simulink model "DiscreteSF_obs"  (R2019b)
settings: Solver=VariableStepAuto  StartTime=0.0  StopTime=10.0  RelTol=1e-3
values from neighbouring files (symbols this model uses):
  th1 = 0.85    [AP_TimeDelay.m]    (also in SmithControl.m; TimeDelayParameters.m = 0.32; positivity_matrix.m; rscale.m)
  th2 = 50    [AP_TimeDelay.m]    (also in SmithControl.m; TimeDelayParameters.m; positivity_matrix.m; rscale.m)
  th3 = 60    [AP_TimeDelay.m]    (also in SmithControl.m; TimeDelayParameters.m = 70; positivity_matrix.m; rscale.m)
undefined symbols (not defined in the file or in its folder): A3, B3, C_obs, D_obs, F3, L_obs
libraries: dspsrcs4 x1
settings Model: Creator=akshita_jain  LastModifiedBy=akshita_jain

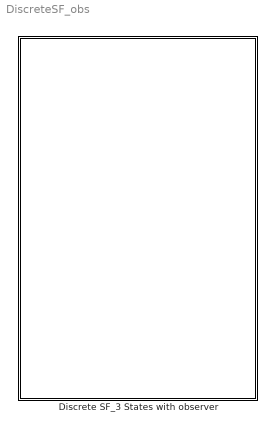
== system DiscreteSF_obs ==
  Discrete SF_3 States with observer : Subsystem

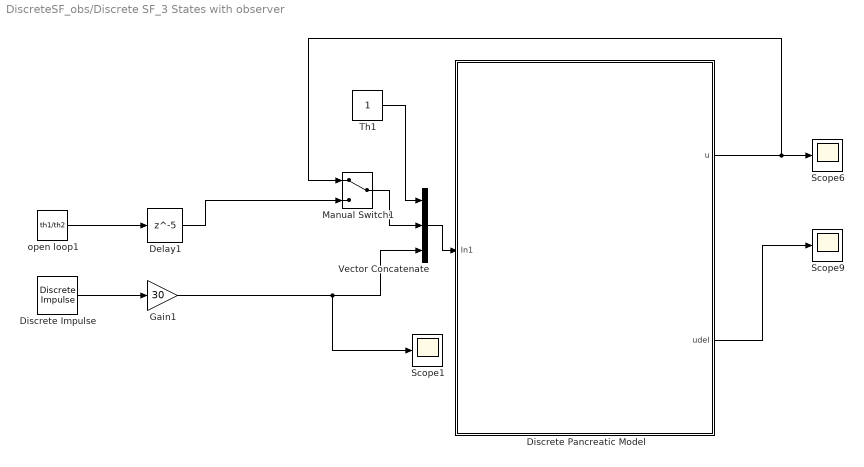
== system DiscreteSF_obs/Discrete SF_3 States with observer ==
  Delay1 : Delay  DelayLength=5  InitialCondition=th1/th2
  Discrete Impulse : dspsrcs4/Discrete  Impulse  Delay=110  SampleTime=1  FrameSample=1  OutputFrames=off  dataType=double  isSigned=on  wordLen=16  udDataType=sfix(16)  fracBitsMode=Best precision  numFracBits=15  OutDataTypeStr=double  LastOutDataTypeStr=double
  Discrete Pancreatic Model : Subsystem
  Gain1 : Gain  Gain=30
  Manual Switch1 : ManualSwitch
  Scope1 : Scope
  Scope6 : Scope
  Scope9 : Scope
  Th1 : Constant
  Vector Concatenate : Concatenate  NumInputs=3
  open loop1 : Constant  Value=th1/th2
  wires:
  Discrete Pancreatic Model/2(udel) -> Scope9/1
  open loop1/1 -> Delay1/1
  Th1/1 -> Vector Concatenate/1
  Vector Concatenate/1 -> Discrete Pancreatic Model/1(In1)
  Gain1/1 -> Scope1/1, Vector Concatenate/3
  Delay1/1 -> Manual Switch1/2
  Manual Switch1/1 -> Vector Concatenate/2
  Discrete Impulse/1 -> Gain1/1
  Discrete Pancreatic Model/1(u) -> Manual Switch1/1, Scope6/1

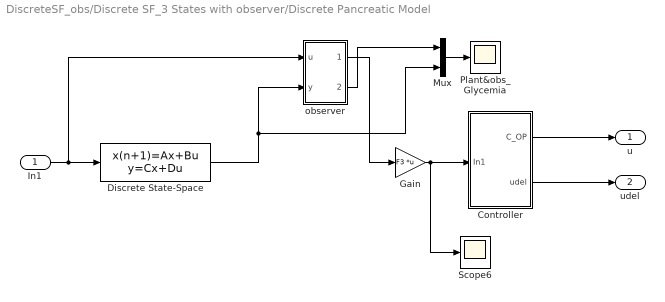
== system DiscreteSF_obs/Discrete SF_3 States with observer/Discrete Pancreatic Model ==
  In1 : Inport
  "Controller " : Subsystem
  Discrete State-Space : DiscreteStateSpace  A=A3  B=B3  C=C_obs  D=D_obs  InitialCondition=[110; th1/th2; 0]  SampleTime=-1  StateName=Glycemia
  Gain : Gain  Gain=F3  Multiplication=Matrix(K*u)
  Mux : Mux  Inputs=2
  Plant&obs_Glycemia : Scope
  Scope6 : Scope
  observer : Subsystem
  u : Outport
  udel : Outport  Port=2
  wires:
  "Controller "/1(C_OP) -> u/1
  "Controller "/2(udel) -> udel/1
  Discrete State-Space/1 -> Mux/2, observer/2(y)
  Gain/1 -> Scope6/1, "Controller "/1(In1)
  In1/1 -> observer/1(u), Discrete State-Space/1
  observer/1(xhat) -> Gain/1
  Mux/1 -> Plant&obs_Glycemia/1
  observer/2(yhat) -> Mux/1

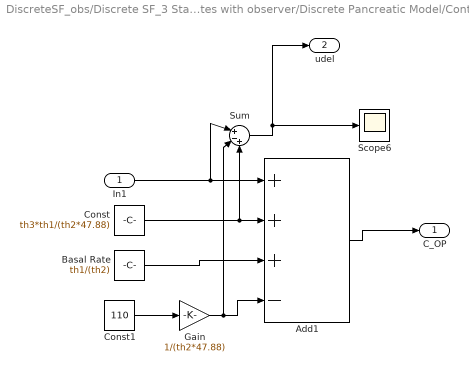
== system DiscreteSF_obs/Discrete SF_3 States with observer/Discrete Pancreatic Model/Controller  ==
  In1 : Inport
  Add1 : Sum  Inputs=+++-
  Basal Rate : Constant  Value=th1/(th2)  VectorParams1D=off
  Const : Constant  Value=th3*th1/(th2*47.88)  VectorParams1D=off
  Const1 : Constant  Value=110  VectorParams1D=off
  Gain : Gain  Gain=1/(th2*47.88)
  Scope6 : Scope
  Sum : Sum  Inputs=|+-+
  C_OP : Outport
  udel : Outport  Port=2
  wires:
  Const/1 -> Sum/3, Add1/2
  Basal Rate/1 -> Add1/3
  Add1/1 -> C_OP/1
  Sum/1 -> Scope6/1, udel/1
  In1/1 -> Sum/1, Add1/1
  Const1/1 -> Gain/1
  Gain/1 -> Sum/2, Add1/4

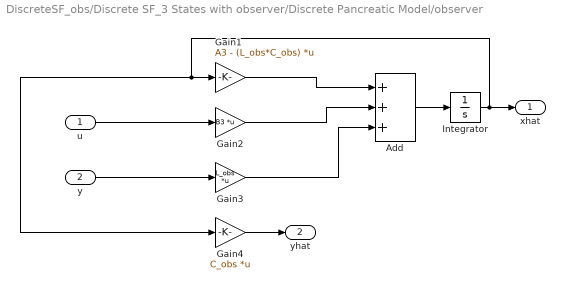
== system DiscreteSF_obs/Discrete SF_3 States with observer/Discrete Pancreatic Model/observer ==
  u : Inport
  y : Inport  Port=2
  Add : Sum  Inputs=3
  Gain1 : Gain  Gain=A3 - (L_obs*C_obs)  Multiplication=Matrix(K*u)
  Gain2 : Gain  Gain=B3  Multiplication=Matrix(K*u)
  Gain3 : Gain  Gain=L_obs  Multiplication=Matrix(K*u)
  Gain4 : Gain  Gain=C_obs  Multiplication=Matrix(K*u)
  Integrator : Integrator  InitialCondition=[110; th1/th2; 0]
  xhat : Outport
  yhat : Outport  Port=2
  wires:
  y/1 -> Gain3/1
  u/1 -> Gain2/1
  Gain1/1 -> Add/1
  Gain2/1 -> Add/2
  Gain3/1 -> Add/3
  Add/1 -> Integrator/1
  Integrator/1 -> Gain1/1, Gain4/1, xhat/1
  Gain4/1 -> yhat/1
